simulink model "new_topavalon"  (Simulink 7.6)
settings: Solver=FixedStepDiscrete  StartTime=0.0  StopTime=100.0  FixedStep=1  RelTol=1e-3
InitFcn:
  | %% DSPBuilder Start
  | alt_dspbuilder_update_model(bdroot)
  | %% DSPBuilder End
undefined symbols (not defined in the file): Pin_AB6, Pin_AE3, Pin_G3, Pin_G4, Pin_H3, Pin_H4, Pin_J5, Pin_J6, Pin_K1, Pin_K2, Pin_L1, Pin_L2, Pin_L3, Pin_L4, Pin_M7, Pin_M8, Pin_N3, Pin_N4, Pin_P1, Pin_P2, Pin_R3, Pin_R4, Pin_R6, Pin_R7, Pin_T3, Pin_T4, Pin_V3, Pin_V4
libraries: allblocks_alteradspbuilder2 x30, Cyclone_III_EP3C120_alteradspbuilder2 x3, simulink x2
settings Model: Creator=DOLSEN  LastModifiedBy=akarapet
settings DataIOCC: SignalLoggingName=sigsOut
settings OptimizationCC: BlockReduction=off  BooleanDataType=off  InitFltsAndDblsToZero=on
settings DebuggingCC: AlgebraicLoopMsg=none  SaveWithParameterizedLinksMsg=none  SignalResolutionControl=TryResolveAllWithWarning  SolverPrmCheckMsg=none  MultiTaskDSMMsg=warning  MultiTaskCondExecSysMsg=none  StrictBusMsg=Warning
settings HardwareCC: TargetUnknown=on
settings RTWCC: IncludeERTFirstTime=on
settings GRTTargetCC: TargetFcnLib=ansi_tfl_tmw.mat  ModelReferenceCompliant=off  MatFileLogging=off

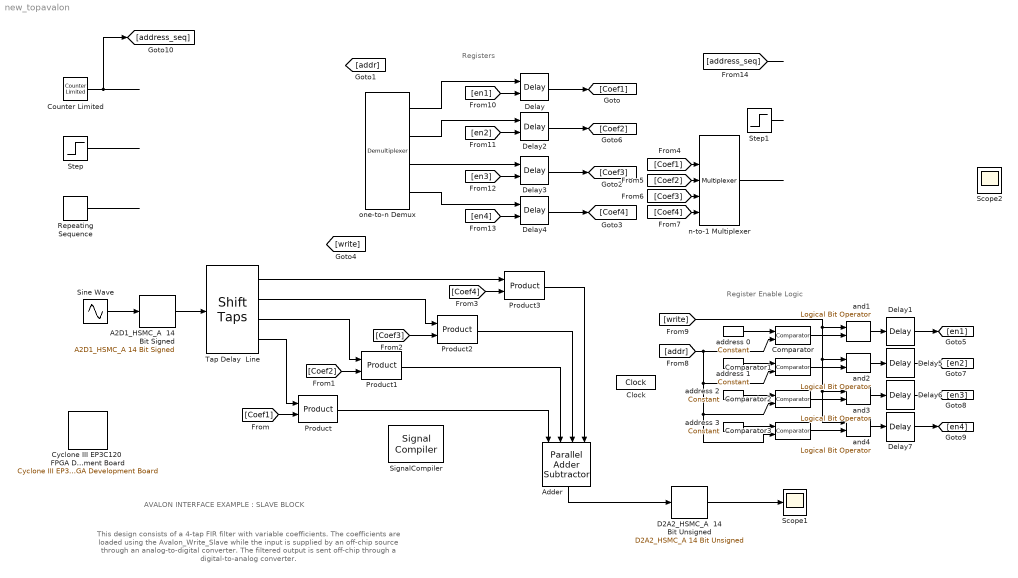
== system new_topavalon ==
  note: AVALON INTERFACE EXAMPLE : SLAVE BLOCK
  note: This design consists of a 4-tap FIR filter with variable coefficients.  The
      | coefficients are loaded using the Avalon_Write_Slave while the input is
      | supplied by an off-chip source through an analog-to-digital converter. The
      | filtered output is sent off-chip through a digital-to-analog converter.
  note: Register Enable Logic
  note: Registers
  A2D1_HSMC_A  14 Bit Signed : Cyclone_III_EP3C120_alteradspbuilder2/A2D1_HSMC_A 14 Bit Signed  iofile=/data/akarapet/qshell_linux64_test/p4/dsp_builder/dsp_builder2/Documentation/DesignExamples/Tutorials/SOPCBuilder/SOPCBlock/tb_new_topavalon/new%5Ftopavalon_A2D1%5FHSMC%5FA+%0A14+Bit+Signed.salt  externalType=Inferred  SpecifyClock=off  location=Pin_P1,Pin_P2,Pin_M7,Pin_M8,Pin_R4,Pin_R3,Pin_T3,Pin_T4,Pin_V3,Pin_V4,Pin_R6,Pin_R7,Pin_AE3,Pin_AB6
  Adder : allblocks_alteradspbuilder2/Parallel Adder Subtractor  number_of_inputs=4  direction=++  use_pipeline=off  pipeline_display=0  phase_selection=1  use_ena=off  use_aclr=off  allowFloatingPointOverride=on  logOutputs=off  logFile=/data/akarapet/qshell_linux64_test/p4/dsp_builder/dsp_builder2/Documentation/DesignExamples/Tutorials/SOPCBuilder/SOPCBlock/tb_new_topavalon/new%5Ftopavalon_Adder.fixedpointlog
  Clock : allblocks_alteradspbuilder2/Clock  ClockPeriod=100  ClockPeriodUnit=ns  SampleTime=1  ResetLatency=0  ResetRegisterCascadeDepth=0  SimulationStartCycle=5  PhaseOffset=0  Reset=aclr  ResetType=Active Low  Export=off
  Comparator : allblocks_alteradspbuilder2/Comparator  direction=a == b  pipeline_display=0  allowFloatingPointOverride=on  logOutputs=off  logFile=/data/akarapet/qshell_linux64_test/p4/dsp_builder/dsp_builder2/Documentation/DesignExamples/Tutorials/SOPCBuilder/SOPCBlock/tb_new_topavalon/new%5Ftopavalon_Comparator.fixedpointlog
  Comparator1 : allblocks_alteradspbuilder2/Comparator  direction=a == b  pipeline_display=0  allowFloatingPointOverride=on  logOutputs=off  logFile=/data/akarapet/qshell_linux64_test/p4/dsp_builder/dsp_builder2/Documentation/DesignExamples/Tutorials/SOPCBuilder/SOPCBlock/tb_new_topavalon/new%5Ftopavalon_Comparator1.fixedpointlog
  Comparator2 : allblocks_alteradspbuilder2/Comparator  direction=a == b  pipeline_display=0  allowFloatingPointOverride=on  logOutputs=off  logFile=/data/akarapet/qshell_linux64_test/p4/dsp_builder/dsp_builder2/Documentation/DesignExamples/Tutorials/SOPCBuilder/SOPCBlock/tb_new_topavalon/new%5Ftopavalon_Comparator2.fixedpointlog
  Comparator3 : allblocks_alteradspbuilder2/Comparator  direction=a == b  pipeline_display=0  allowFloatingPointOverride=on  logOutputs=off  logFile=/data/akarapet/qshell_linux64_test/p4/dsp_builder/dsp_builder2/Documentation/DesignExamples/Tutorials/SOPCBuilder/SOPCBlock/tb_new_topavalon/new%5Ftopavalon_Comparator3.fixedpointlog
  Counter Limited : simulink/Sources/Counter Limited  SystemSampleTime=-1  uplimit=3  tsamp=1
  Cyclone III EP3C120  FPGA Development Board : Cyclone_III_EP3C120_alteradspbuilder2/Cyclone III EP3C120 FPGA Development Board  ClockPinIn=Pin_AH15  GlobalResetPin=Pin_T21  device=EP3C120F780C7
  D2A2_HSMC_A  14 Bit Unsigned : Cyclone_III_EP3C120_alteradspbuilder2/D2A2_HSMC_A 14 Bit Unsigned  iofile=/data/akarapet/qshell_linux64_test/p4/dsp_builder/dsp_builder2/Documentation/DesignExamples/Tutorials/SOPCBuilder/SOPCBlock/tb_new_topavalon/new%5Ftopavalon_D2A2%5FHSMC%5FA+%0A14+Bit+Unsigned.capture  externalType=Inferred  location=Pin_G3,Pin_G4,Pin_H3,Pin_H4,Pin_J5,Pin_J6,Pin_K1,Pin_K2,Pin_L1,Pin_L2,Pin_L3,Pin_L4,Pin_N3,Pin_N4
  Delay : allblocks_alteradspbuilder2/Delay  pipeline=1  pipeline_display=1  ClockPhase=1  use_ena=on  use_sclr=off  allowFloatingPointOverride=on  logOutputs=off  logFile=/data/akarapet/qshell_linux64_test/p4/dsp_builder/dsp_builder2/Documentation/DesignExamples/Tutorials/SOPCBuilder/SOPCBlock/tb_new_topavalon/new%5Ftopavalon_Delay.fixedpointlog  use_init=off  reset_value=1
  Delay1 : allblocks_alteradspbuilder2/Delay  pipeline=1  pipeline_display=1  ClockPhase=1  use_ena=off  use_sclr=off  allowFloatingPointOverride=on  logOutputs=off  logFile=/data/akarapet/qshell_linux64_test/p4/dsp_builder/dsp_builder2/Documentation/DesignExamples/Tutorials/SOPCBuilder/SOPCBlock/tb_new_topavalon/new%5Ftopavalon_Delay1.fixedpointlog  use_init=off  reset_value=1
  Delay2 : allblocks_alteradspbuilder2/Delay  pipeline=1  pipeline_display=1  ClockPhase=1  use_ena=on  use_sclr=off  allowFloatingPointOverride=on  logOutputs=off  logFile=/data/akarapet/qshell_linux64_test/p4/dsp_builder/dsp_builder2/Documentation/DesignExamples/Tutorials/SOPCBuilder/SOPCBlock/tb_new_topavalon/new%5Ftopavalon_Delay2.fixedpointlog  use_init=off  reset_value=1
  Delay3 : allblocks_alteradspbuilder2/Delay  pipeline=1  pipeline_display=1  ClockPhase=1  use_ena=on  use_sclr=off  allowFloatingPointOverride=on  logOutputs=off  logFile=/data/akarapet/qshell_linux64_test/p4/dsp_builder/dsp_builder2/Documentation/DesignExamples/Tutorials/SOPCBuilder/SOPCBlock/tb_new_topavalon/new%5Ftopavalon_Delay3.fixedpointlog  use_init=off  reset_value=1
  Delay4 : allblocks_alteradspbuilder2/Delay  pipeline=1  pipeline_display=1  ClockPhase=1  use_ena=on  use_sclr=off  allowFloatingPointOverride=on  logOutputs=off  logFile=/data/akarapet/qshell_linux64_test/p4/dsp_builder/dsp_builder2/Documentation/DesignExamples/Tutorials/SOPCBuilder/SOPCBlock/tb_new_topavalon/new%5Ftopavalon_Delay4.fixedpointlog  use_init=off  reset_value=1
  Delay5 : allblocks_alteradspbuilder2/Delay  pipeline=1  pipeline_display=1  ClockPhase=1  use_ena=off  use_sclr=off  allowFloatingPointOverride=on  logOutputs=off  logFile=/data/akarapet/qshell_linux64_test/p4/dsp_builder/dsp_builder2/Documentation/DesignExamples/Tutorials/SOPCBuilder/SOPCBlock/tb_new_topavalon/new%5Ftopavalon_Delay5.fixedpointlog  use_init=off  reset_value=1
  Delay6 : allblocks_alteradspbuilder2/Delay  pipeline=1  pipeline_display=1  ClockPhase=1  use_ena=off  use_sclr=off  allowFloatingPointOverride=on  logOutputs=off  logFile=/data/akarapet/qshell_linux64_test/p4/dsp_builder/dsp_builder2/Documentation/DesignExamples/Tutorials/SOPCBuilder/SOPCBlock/tb_new_topavalon/new%5Ftopavalon_Delay6.fixedpointlog  use_init=off  reset_value=1
  Delay7 : allblocks_alteradspbuilder2/Delay  pipeline=1  pipeline_display=1  ClockPhase=1  use_ena=off  use_sclr=off  allowFloatingPointOverride=on  logOutputs=off  logFile=/data/akarapet/qshell_linux64_test/p4/dsp_builder/dsp_builder2/Documentation/DesignExamples/Tutorials/SOPCBuilder/SOPCBlock/tb_new_topavalon/new%5Ftopavalon_Delay7.fixedpointlog  use_init=off  reset_value=1
  Product : allblocks_alteradspbuilder2/Product  BusType=Inferred  bwl=8  bwr=0  pipeline=0  pipeline_display=0  phase_selection=1  use_ena=off  use_aclr=off  UseLPM=off  UseDedicatedCircuitry=off  allowFloatingPointOverride=on  logOutputs=off  logFile=/data/akarapet/qshell_linux64_test/p4/dsp_builder/dsp_builder2/Documentation/DesignExamples/Tutorials/SOPCBuilder/SOPCBlock/tb_new_topavalon/new%5Ftopavalon_Product.fixedpointlog
  Product1 : allblocks_alteradspbuilder2/Product  BusType=Inferred  bwl=8  bwr=0  pipeline=0  pipeline_display=0  phase_selection=1  use_ena=off  use_aclr=off  UseLPM=off  UseDedicatedCircuitry=off  allowFloatingPointOverride=on  logOutputs=off  logFile=/data/akarapet/qshell_linux64_test/p4/dsp_builder/dsp_builder2/Documentation/DesignExamples/Tutorials/SOPCBuilder/SOPCBlock/tb_new_topavalon/new%5Ftopavalon_Product1.fixedpointlog
  Product2 : allblocks_alteradspbuilder2/Product  BusType=Inferred  bwl=8  bwr=0  pipeline=0  pipeline_display=0  phase_selection=1  use_ena=off  use_aclr=off  UseLPM=off  UseDedicatedCircuitry=off  allowFloatingPointOverride=on  logOutputs=off  logFile=/data/akarapet/qshell_linux64_test/p4/dsp_builder/dsp_builder2/Documentation/DesignExamples/Tutorials/SOPCBuilder/SOPCBlock/tb_new_topavalon/new%5Ftopavalon_Product2.fixedpointlog
  Product3 : allblocks_alteradspbuilder2/Product  BusType=Inferred  bwl=8  bwr=0  pipeline=0  pipeline_display=0  phase_selection=1  use_ena=off  use_aclr=off  UseLPM=off  UseDedicatedCircuitry=off  allowFloatingPointOverride=on  logOutputs=off  logFile=/data/akarapet/qshell_linux64_test/p4/dsp_builder/dsp_builder2/Documentation/DesignExamples/Tutorials/SOPCBuilder/SOPCBlock/tb_new_topavalon/new%5Ftopavalon_Product3.fixedpointlog
  Repeating Sequence : simulink/Sources/Repeating Sequence  SystemSampleTime=-1  rep_seq_t=[0 1 2 3 4]  rep_seq_y=[1 0 0 0 0]
  Scope1 : Scope
      settings: SampleInput=on
  Scope2 : Scope
      settings: SampleInput=on
  SignalCompiler : allblocks_alteradspbuilder2/Signal Compiler  DeviceFamily=Stratix II  DeviceName=EP2S60F1020C4ES  EnableSignalTap=off  SignalTapDepth=128  UseBoardBlock=off  StpUseDefaultClock=on  StpClock=Clock  ExportDir=C:\Documents and Settings\sichou\My Documents
  Sine Wave : Sin  Amplitude=2^11-1  SampleTime=1
  Step : Step  Time=4  Before=1  After=0  SampleTime=1
  Step1 : Step  Time=10  Before=1  After=0  SampleTime=1
  Tap Delay  Line : allblocks_alteradspbuilder2/Shift Taps  number_of_taps=4  tap_distance=1  use_shiftout=off  use_ena=off  use_sclr=off  use_dedicated_circuitry=on  ram_type=AUTO  allowFloatingPointOverride=on  logOutputs=off  logFile=/data/akarapet/qshell_linux64_test/p4/dsp_builder/dsp_builder2/Documentation/DesignExamples/Tutorials/SOPCBuilder/SOPCBlock/tb_new_topavalon/new%5Ftopavalon_Tap+Delay+%0ALine%3A%3At.fixedpointlog,/data/akarapet/qshell_linux64_test/p4/dsp_builder/dsp_builder2/Documentation/DesignExamples/Tutorials/SOPCBuilder/SOPCBlock/tb_new_topavalon/new%5Ftopavalon_Tap+Delay+%0ALine%3A%3At.fixedpointlog,/data/akarapet/qshell_linux64_test/p4/dsp_builder/dsp_builder2/Documentation/DesignExamples/Tutorials/SOPCBuilder/SOPCBlock/tb_new_topavalon/new%5Ftopavalon_Tap+Delay+%0ALine%3A%3At.fixedpointlog,/data/akarapet/qshell_linux64_test/p4/dsp_builder/dsp_builder2/Documentation/DesignExamples/Tutorials/SOPCBuilder/SOPCBlock/tb_new_topavalon/new%5Ftopavalon_Tap+Delay+%0ALine%3A%3At.fixedpointlog,
  address 0 : allblocks_alteradspbuilder2/Constant  mask_cst=0  BusType=Unsigned Integer  bwl=2  bwr=0  roundMode=Truncate  satMode=Wrap  SpecifyClock=off  allowFloatingPointOverride=on  logOutputs=off  logFile=/data/akarapet/qshell_linux64_test/p4/dsp_builder/dsp_builder2/Documentation/DesignExamples/Tutorials/SOPCBuilder/SOPCBlock/tb_new_topavalon/new%5Ftopavalon_address+0.fixedpointlog
  address 1 : allblocks_alteradspbuilder2/Constant  mask_cst=1  BusType=Unsigned Integer  bwl=2  bwr=0  roundMode=Truncate  satMode=Wrap  SpecifyClock=off  allowFloatingPointOverride=on  logOutputs=off  logFile=/data/akarapet/qshell_linux64_test/p4/dsp_builder/dsp_builder2/Documentation/DesignExamples/Tutorials/SOPCBuilder/SOPCBlock/tb_new_topavalon/new%5Ftopavalon_address+1.fixedpointlog
  address 2 : allblocks_alteradspbuilder2/Constant  mask_cst=2  BusType=Unsigned Integer  bwl=2  bwr=0  roundMode=Truncate  satMode=Wrap  SpecifyClock=off  allowFloatingPointOverride=on  logOutputs=off  logFile=/data/akarapet/qshell_linux64_test/p4/dsp_builder/dsp_builder2/Documentation/DesignExamples/Tutorials/SOPCBuilder/SOPCBlock/tb_new_topavalon/new%5Ftopavalon_address+2.fixedpointlog
  address 3 : allblocks_alteradspbuilder2/Constant  mask_cst=3  BusType=Unsigned Integer  bwl=2  bwr=0  roundMode=Truncate  satMode=Wrap  SpecifyClock=off  allowFloatingPointOverride=on  logOutputs=off  logFile=/data/akarapet/qshell_linux64_test/p4/dsp_builder/dsp_builder2/Documentation/DesignExamples/Tutorials/SOPCBuilder/SOPCBlock/tb_new_topavalon/new%5Ftopavalon_address+3.fixedpointlog
  and{1..4} (4 alike) : allblocks_alteradspbuilder2/Logical Bit Operator  LogicalOperator=AND  user_inputs=2  pipeline_display=0
  n-to-1 Multiplexer : allblocks_alteradspbuilder2/Multiplexer  numInputs=4  pipeline=0  oneHot=off  pipeline_display=0  use_ena=off  use_aclr=off  allowFloatingPointOverride=on  logOutputs=off  logFile=/data/akarapet/qshell_linux64_test/p4/dsp_builder/dsp_builder2/Documentation/DesignExamples/Tutorials/SOPCBuilder/SOPCBlock/tb_new_topavalon/new%5Ftopavalon_n-to-1+Multiplexer.fixedpointlog
  one-to-n Demux : allblocks_alteradspbuilder2/Demultiplexer  numOutputs=4  pipeline_display=1  use_ena=on  use_sclr=off  allowFloatingPointOverride=on  logOutputs=off  logFile=/new%5Ftopavalon_one-to-n+Demux%3A%3Aq.fixedpointlog,/new%5Ftopavalon_one-to-n+Demux%3A%3Aq.fixedpointlog,/new%5Ftopavalon_one-to-n+Demux%3A%3Aq.fixedpointlog,/new%5Ftopavalon_one-to-n+Demux%3A%3Aq.fixedpointlog,
  wires:
  Tap Delay  Line/4 -> Product/1
  Tap Delay  Line/3 -> Product1/1
  Tap Delay  Line/2 -> Product2/1
  Tap Delay  Line/1 -> Product3/1
  Product/1 -> Adder/1
  A2D1_HSMC_A  14 Bit Signed/1 -> Tap Delay  Line/1
  Product1/1 -> Adder/2
  Product2/1 -> Adder/3
  Product3/1 -> Adder/4
  Adder/1 -> D2A2_HSMC_A  14 Bit Unsigned/1
  [Coef1] -> Product/2
  [Coef2] -> Product1/2
  [Coef3] -> Product2/2
  [Coef4] -> Product3/2
  one-to-n Demux/1 -> Delay/1
  one-to-n Demux/2 -> Delay2/1
  one-to-n Demux/3 -> Delay3/1
  one-to-n Demux/4 -> Delay4/1
  ? -> one-to-n Demux/2, [addr]
  ? -> one-to-n Demux/3, [write]
  ? -> one-to-n Demux/1
  n-to-1 Multiplexer/1 -> ?
  Sine Wave/1 -> A2D1_HSMC_A  14 Bit Signed/1
  Delay/1 -> [Coef1]
  Delay2/1 -> [Coef2]
  Delay3/1 -> [Coef3]
  Delay4/1 -> [Coef4]
  address 0/1 -> Comparator/1
  address 1/1 -> Comparator1/1
  address 2/1 -> Comparator2/1
  address 3/1 -> Comparator3/1
  Comparator/1 -> and1/2
  Comparator1/1 -> and2/2
  Comparator2/1 -> and3/2
  Comparator3/1 -> and4/2
  [write] -> and3/1, and4/1, and2/1, and1/1
  and1/1 -> Delay1/1
  and2/1 -> Delay5/1
  and3/1 -> Delay6/1
  and4/1 -> Delay7/1
  [en1] -> Delay/2
  [en2] -> Delay2/2
  [en3] -> Delay3/2
  [en4] -> Delay4/2
  Delay1/1 -> [en1]
  Delay5/1 -> [en2]
  Delay6/1 -> [en3]
  Delay7/1 -> [en4]
  [addr] -> Comparator/2, Comparator1/2, Comparator2/2, Comparator3/2
  D2A2_HSMC_A  14 Bit Unsigned/1 -> Scope1/1
  ? -> n-to-1 Multiplexer/1
  [Coef1] -> n-to-1 Multiplexer/2
  [Coef2] -> n-to-1 Multiplexer/3
  [Coef3] -> n-to-1 Multiplexer/4
  [Coef4] -> n-to-1 Multiplexer/5
  Counter Limited/1 -> [address_seq]
  Step/1 -> ?
  Repeating Sequence/1 -> ?
  ? -> Scope2/1
  [address_seq] -> ?
  Step1/1 -> ?
